simulink model "Angular_Frame_Conversion_to_Inertia"  (R2018a)
settings: Solver=VariableStepAuto  StartTime=0.0  StopTime=10.0  RelTol=1e-3
settings Model: Creator=Ibrahim  LastModifiedBy=Ibrahim

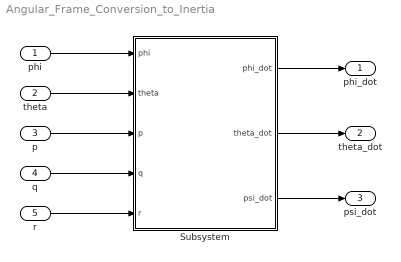
== system Angular_Frame_Conversion_to_Inertia ==
  phi : Inport
  theta : Inport  Port=2
  p : Inport  Port=3
  q : Inport  Port=4
  r : Inport  Port=5
  Subsystem : Subsystem
  phi_dot : Outport
  theta_dot : Outport  Port=2
  psi_dot : Outport  Port=3
  wires:
  phi/1 -> Subsystem/1(phi)
  theta/1 -> Subsystem/2(theta)
  p/1 -> Subsystem/3(p)
  q/1 -> Subsystem/4(q)
  r/1 -> Subsystem/5(r)
  Subsystem/1(phi_dot) -> phi_dot/1
  Subsystem/2(theta_dot) -> theta_dot/1
  Subsystem/3(psi_dot) -> psi_dot/1

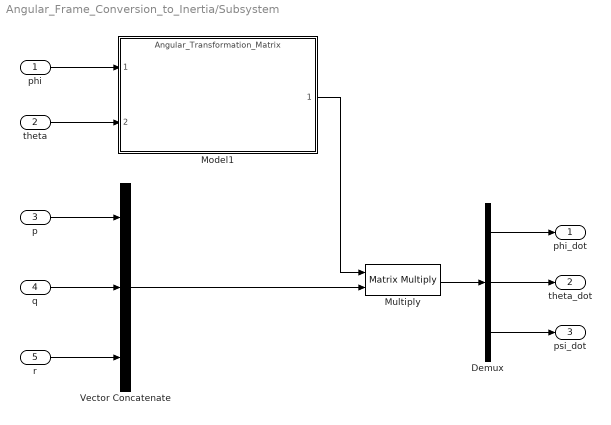
== system Angular_Frame_Conversion_to_Inertia/Subsystem ==
  phi : Inport
  theta : Inport  Port=2
  p : Inport  Port=3
  q : Inport  Port=4
  r : Inport  Port=5
  Demux : Demux  Outputs=3
  Model1 : ModelReference  ModelNameDialog=Angular_Transformation_Matrix.slx  SimulationMode=Normal  ModelReferenceVersion=1.5
  Multiply : Product  Multiplication=Matrix(*)
  Vector Concatenate : Concatenate  NumInputs=3
  phi_dot : Outport
  theta_dot : Outport  Port=2
  psi_dot : Outport  Port=3
  wires:
  Vector Concatenate/1 -> Multiply/2
  Multiply/1 -> Demux/1
  Demux/2 -> theta_dot/1
  Demux/1 -> phi_dot/1
  r/1 -> Vector Concatenate/3
  theta/1 -> Model1/2
  q/1 -> Vector Concatenate/2
  Demux/3 -> psi_dot/1
  phi/1 -> Model1/1
  p/1 -> Vector Concatenate/1
  Model1/1 -> Multiply/1
